simulink model "FP_Solutions_Part_3_disturbance"  (R2024b)
settings: Solver=VariableStepAuto  StartTime=0.0  StopTime=tspan  FixedStep=10  RelTol=1e-8
model workspace (MATLAB code in the model file):
  | mu = 398601; % km
  | Re = 6378.137; %km
values from neighbouring files (symbols this model uses):
  E_b_LVLH_0 = [phi_0; theta_0; psi_0]    [FP_Solution_Part_3.m]
  J = (Bus_I - Bus_m*skew(r_Bus)*skew(r_Bus)) +     (Sensor_I - Sensor_m*skew(r_Sensor)*skew(r_Sensor)) +      (Sp_minus_I - Sp_minus_m*skew(r_Sp_minus)*skew(r_Sp_minus)) +     (Sp_plus_I - Sp_plus_m*skew(r_Sp_plus)*skew(r_Sp_plus))    [FP_Solution_Part_3.m]
  JD_0 = 2460390    [FP_Solution_Part_3.m]
  q_b_LVLH_0 = [0; 0; 0; 1]    [FP_Solution_Part_3.m]
  residual_dipole_moment = [0;0;-0.5]    [FP_Solution_Part_3.m]
  Sun_vec = [1;0;0]    [FP_Solution_Part_3.m]
  surfaceProperties = [Areas rhos normals]    [FP_Solution_Part_3.m]
  T_c = [0; 0; 0]    [FP_Solution_Part_3.m]
undefined symbols (not defined in the file or in its folder): r_ECI_0, v_ECI_0
settings Model: Creator=emehiel  LastModifiedBy=nicho
settings SolverCC: AlgebraicLoopSolver=TrustRegion
settings DebuggingCC: UnconnectedInputMsg=warning  UnconnectedOutputMsg=warning  UnconnectedLineMsg=warning
settings ModelReferenceCC: EnableRefExpFcnMdlSchedulingChecks=on
settings RTWCC: GPUComputeCapability=3.5

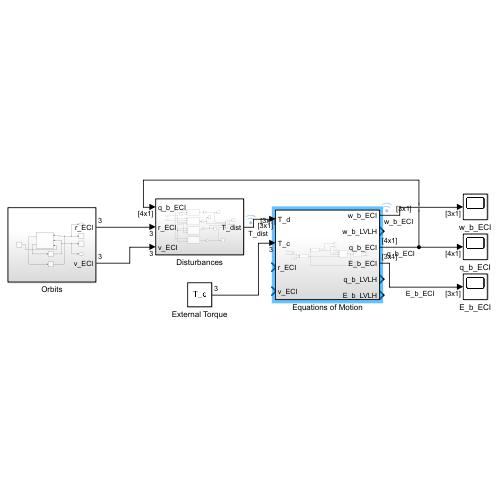
[thumbnail: Simulink's stored preview of the top-level diagram]
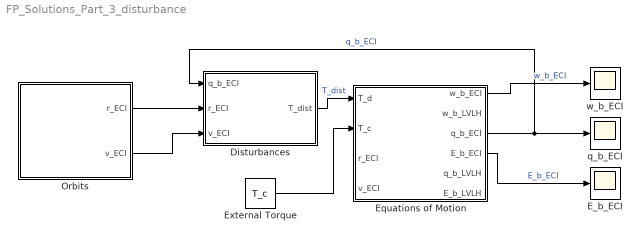
== system FP_Solutions_Part_3_disturbance ==
  Disturbances : Subsystem
  E_b_ECI : Scope
  Equations of Motion : Subsystem
  External Torque : Constant  Value=T_c
  Orbits : Subsystem
  q_b_ECI : Scope
  w_b_ECI : Scope
  wires:
  Orbits/1(r_ECI) -> Disturbances/2(r_ECI)
  Orbits/2(v_ECI) -> Disturbances/3(v_ECI)
  Equations of Motion/3(q_b_ECI) -> Disturbances/1(q_b_ECI), q_b_ECI/1  "q_b_ECI"
  Equations of Motion/1(w_b_ECI) -> w_b_ECI/1  "w_b_ECI"
  Disturbances/1(T_dist) -> Equations of Motion/1(T_d)  "T_dist"
  Equations of Motion/4(E_b_ECI) -> E_b_ECI/1  "E_b_ECI"
  External Torque/1 -> Equations of Motion/2(T_c)

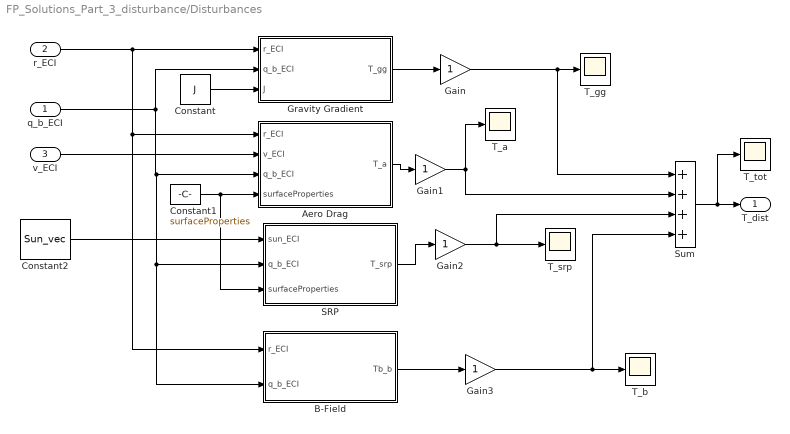
== system FP_Solutions_Part_3_disturbance/Disturbances ==
  q_b_ECI : Inport  PortDimensions=[4 1]
  r_ECI : Inport  Port=2
  v_ECI : Inport  Port=3
  Aero Drag : MATLAB Function  TreatAsAtomicUnit=on
  B-Field : Subsystem
  Constant : Constant  Value=J
  Constant1 : Constant  Value=surfaceProperties
  Constant2 : Constant  Value=Sun_vec
  Gain{,1..3} (4 alike) : Gain
  Gravity Gradient : MATLAB Function  TreatAsAtomicUnit=on
  SRP : MATLAB Function  TreatAsAtomicUnit=on
  Sum : Sum  Inputs=++++
  T_a : Scope
  T_b : Scope
  T_gg : Scope
  T_srp : Scope
  T_tot : Scope
  T_dist : Outport
  wires:
  Sum/1 -> T_tot/1, T_dist/1
  Aero Drag/1(T_a) -> Gain1/1
  Gravity Gradient/1(T_gg) -> Gain/1
  SRP/1(T_srp) -> Gain2/1
  Constant1/1 -> SRP/3(surfaceProperties), Aero Drag/4(surfaceProperties)
  v_ECI/1 -> Aero Drag/2(v_ECI)
  q_b_ECI/1 -> B-Field/2(q_b_ECI), SRP/2(q_b_ECI), Aero Drag/3(q_b_ECI), Gravity Gradient/2(q_b_ECI)
  Constant/1 -> Gravity Gradient/3(J)
  Constant2/1 -> SRP/1(sun_ECI)
  r_ECI/1 -> B-Field/1(r_ECI), Aero Drag/1(r_ECI), Gravity Gradient/1(r_ECI)
  B-Field/1(Tb_b) -> Gain3/1
  Gain/1 -> Sum/1, T_gg/1
  Gain1/1 -> Sum/2, T_a/1
  Gain3/1 -> T_b/1, Sum/4
  Gain2/1 -> Sum/3, T_srp/1

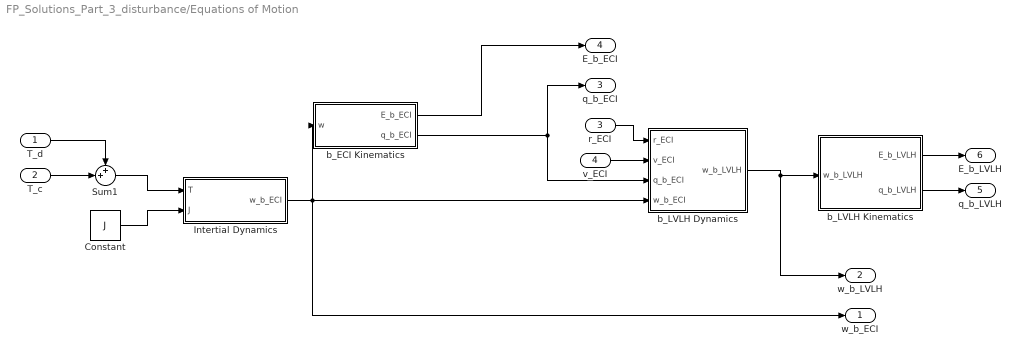
== system FP_Solutions_Part_3_disturbance/Equations of Motion ==
  T_d : Inport
  T_c : Inport  Port=2
  r_ECI : Inport  Port=3
  v_ECI : Inport  Port=4
  Constant : Constant  Value=J
  "Intertial Dynamics " : Subsystem
  Sum1 : Sum  Inputs=++|
  b_ECI Kinematics : Subsystem
  b_LVLH Dynamics : Subsystem
  b_LVLH Kinematics : Subsystem
  w_b_ECI : Outport  VectorParamsAs1DForOutWhenUnconnected=off
  w_b_LVLH : Outport  Port=2  PortDimensions=[3 1]  VectorParamsAs1DForOutWhenUnconnected=off
  q_b_ECI : Outport  Port=3  PortDimensions=[4 1]  VectorParamsAs1DForOutWhenUnconnected=off
  E_b_ECI : Outport  Port=4  PortDimensions=[3 1]  VectorParamsAs1DForOutWhenUnconnected=off
  q_b_LVLH : Outport  Port=5  PortDimensions=[4 1]  VectorParamsAs1DForOutWhenUnconnected=off
  E_b_LVLH : Outport  Port=6  PortDimensions=[3 1]  VectorParamsAs1DForOutWhenUnconnected=off
  wires:
  T_d/1 -> Sum1/1
  T_c/1 -> Sum1/2
  Sum1/1 -> "Intertial Dynamics "/1(T)
  Constant/1 -> "Intertial Dynamics "/2(J)
  b_ECI Kinematics/2(q_b_ECI) -> q_b_ECI/1, b_LVLH Dynamics/3(q_b_ECI)
  b_LVLH Kinematics/2(q_b_LVLH) -> q_b_LVLH/1
  r_ECI/1 -> b_LVLH Dynamics/1("r_ECI ")
  b_LVLH Dynamics/1(w_b_LVLH) -> w_b_LVLH/1, b_LVLH Kinematics/1(w_b_LVLH)
  "Intertial Dynamics "/1(w_b_ECI) -> w_b_ECI/1, b_LVLH Dynamics/4(w_b_ECI), b_ECI Kinematics/1(w)
  b_ECI Kinematics/1(E_b_ECI) -> E_b_ECI/1
  v_ECI/1 -> b_LVLH Dynamics/2(v_ECI)
  b_LVLH Kinematics/1(E_b_LVLH) -> E_b_LVLH/1

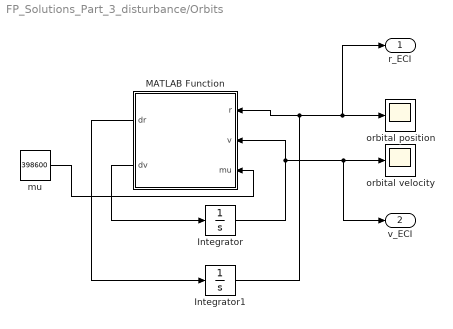
== system FP_Solutions_Part_3_disturbance/Orbits ==
  Integrator : Integrator  InitialCondition=v_ECI_0
  Integrator1 : Integrator  InitialCondition=r_ECI_0
  MATLAB Function : MATLAB Function  TreatAsAtomicUnit=on
  mu : Constant  Value=398600
  orbital position : Scope
  orbital velocity : Scope
  r_ECI : Outport  VectorParamsAs1DForOutWhenUnconnected=off
  v_ECI : Outport  Port=2  VectorParamsAs1DForOutWhenUnconnected=off
  wires:
  Integrator/1 -> v_ECI/1, orbital velocity/1, MATLAB Function/2(v)
  Integrator1/1 -> r_ECI/1, orbital position/1, MATLAB Function/1(r)
  MATLAB Function/1(dr) -> Integrator1/1
  MATLAB Function/2(dv) -> Integrator/1
  mu/1 -> MATLAB Function/3(mu)

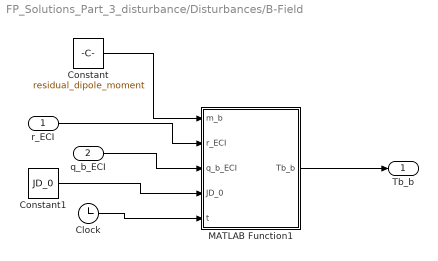
== system FP_Solutions_Part_3_disturbance/Disturbances/B-Field ==
  r_ECI : Inport
  q_b_ECI : Inport  Port=2
  Clock : Clock
  Constant : Constant  Value=residual_dipole_moment  VectorParams1D=off
  Constant1 : Constant  Value=JD_0
  MATLAB Function1 : MATLAB Function  TreatAsAtomicUnit=on
  Tb_b : Outport
  wires:
  MATLAB Function1/1(Tb_b) -> Tb_b/1
  q_b_ECI/1 -> MATLAB Function1/3(q_b_ECI)
  r_ECI/1 -> MATLAB Function1/2(r_ECI)
  Clock/1 -> MATLAB Function1/5(t)
  Constant1/1 -> MATLAB Function1/4(JD_0)
  Constant/1 -> MATLAB Function1/1(m_b)

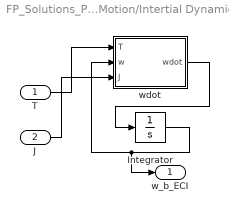
== system FP_Solutions_Part_3_disturbance/Equations of Motion/Intertial Dynamics  ==
  T : Inport
  J : Inport  Port=2
  Integrator : Integrator  InitialCondition=[0.001; -0.001; 0.002]
  wdot : MATLAB Function  TreatAsAtomicUnit=on
  w_b_ECI : Outport
  wires:
  Integrator/1 -> wdot/2(w), w_b_ECI/1
  wdot/1(wdot) -> Integrator/1
  T/1 -> wdot/1(T)
  J/1 -> wdot/3(J)

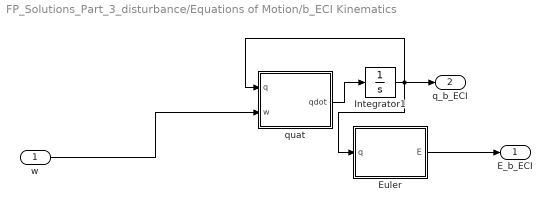
== system FP_Solutions_Part_3_disturbance/Equations of Motion/b_ECI Kinematics ==
  w : Inport
  Euler : MATLAB Function  TreatAsAtomicUnit=on
  Integrator1 : Integrator  InitialCondition=[0;0;0;1]
  quat : MATLAB Function  TreatAsAtomicUnit=on
  E_b_ECI : Outport  VectorParamsAs1DForOutWhenUnconnected=off
  q_b_ECI : Outport  Port=2  VectorParamsAs1DForOutWhenUnconnected=off
  wires:
  w/1 -> quat/2(w)
  Integrator1/1 -> quat/1(q), Euler/1(q), q_b_ECI/1
  quat/1(qdot) -> Integrator1/1
  Euler/1(E) -> E_b_ECI/1

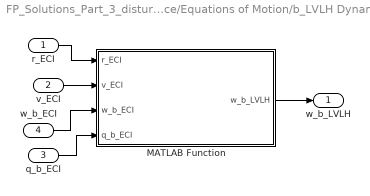
== system FP_Solutions_Part_3_disturbance/Equations of Motion/b_LVLH Dynamics ==
  "r_ECI " : Inport
  v_ECI : Inport  Port=2
  q_b_ECI : Inport  Port=3
  w_b_ECI : Inport  Port=4
  MATLAB Function : MATLAB Function  TreatAsAtomicUnit=on
  w_b_LVLH : Outport  VectorParamsAs1DForOutWhenUnconnected=off
  wires:
  MATLAB Function/1(w_b_LVLH) -> w_b_LVLH/1
  "r_ECI "/1 -> MATLAB Function/1(r_ECI)
  v_ECI/1 -> MATLAB Function/2(v_ECI)
  q_b_ECI/1 -> MATLAB Function/4(q_b_ECI)
  w_b_ECI/1 -> MATLAB Function/3(w_b_ECI)

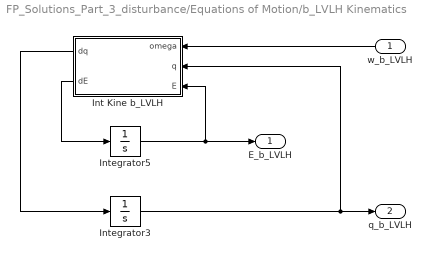
== system FP_Solutions_Part_3_disturbance/Equations of Motion/b_LVLH Kinematics ==
  w_b_LVLH : Inport
  Int Kine b_LVLH : MATLAB Function  TreatAsAtomicUnit=on
  Integrator3 : Integrator  InitialCondition=q_b_LVLH_0
  Integrator5 : Integrator  InitialCondition=E_b_LVLH_0
  E_b_LVLH : Outport  PortDimensions=[3 1]  VectorParamsAs1DForOutWhenUnconnected=off
  q_b_LVLH : Outport  Port=2  VectorParamsAs1DForOutWhenUnconnected=off
  wires:
  Int Kine b_LVLH/1(dq) -> Integrator3/1
  Integrator3/1 -> Int Kine b_LVLH/2(q), q_b_LVLH/1
  Int Kine b_LVLH/2(dE) -> Integrator5/1
  Integrator5/1 -> E_b_LVLH/1, Int Kine b_LVLH/3(E)
  w_b_LVLH/1 -> Int Kine b_LVLH/1(omega)

== matlab function FP_Solutions_Part_3_disturbance/Equations of Motion/b_ECI Kinematics/quat ==
  data: q input; qdot output; w input
function qdot = fcn(q, w)
%#codegen

q = reshape(q,4,1);
w = reshape(w,3,1);

wx = w(1);
wy = w(2);
wz = w(3);

Omega = [  0   -wx  -wy  -wz;
          wx    0    wz  -wy;
          wy   -wz   0    wx;
          wz    wy  -wx   0 ];

qdot = 0.5 * Omega * q;

end

== matlab function FP_Solutions_Part_3_disturbance/Equations of Motion/b_LVLH Dynamics/MATLAB Function ==
  data: r_ECI input; v_ECI input; w_b_ECI input; q_b_ECI input; w_b_LVLH output
function w_b_LVLH = fcn(r_ECI, v_ECI, w_b_ECI, q_b_ECI)
%#codegen

% Compute the angular velocity of LVLH wrt ECI in Body components

rhat = r_ECI / norm(r_ECI);
hvec = cross(r_ECI, v_ECI);
hhat = hvec / norm(hvec);
that = cross(-rhat, hhat);
that = that / norm(that);

C_LVLH_ECI = [hhat.';
                that.';
               (-rhat).'];

q_b_LVLH = circle_cross(transpose(C_LVLH_ECI),q_b_ECI);

w_b_LVLH = w_b_ECI*transpose(C_LVLH_ECI);

== matlab function FP_Solutions_Part_3_disturbance/Disturbances/Gravity Gradient ==
  data: r_ECI input; T_gg output; q_b_ECI input; J input
function T_gg = gg_torque(r_ECI, q_b_ECI, J)
% GG_TORQUE Gravity-gradient torque in body frame
%
% Inputs:
%   r_ECI    3x1 position vector in ECI [km]
%   q_b_ECI  4x1 quaternion [q1;q2;q3;q4], scalar last
%   J        3x3 spacecraft inertia matrix [kg*m^2]
%
% Output:
%   T_gg     3x1 gravity-gradient torque in body frame [N*m]

    mu = 398600;  % km^3/s^2

    r_ECI = r_ECI(:);
    q_b_ECI = q_b_ECI(:);

    r = norm(r_ECI);
    if r == 0
        T_gg = zeros(3,1);
        return
    end

    % Position direction in body frame
    C_b_ECI = quat2C(q_b_ECI);
    r_b = C_b_ECI * r_ECI;
    rhat_b = r_b / norm(r_b);

    % Gravity-gradient torque
    T_gg = (3*mu/r^5) * cross(rhat_b, J*rhat_b);
end

== matlab function FP_Solutions_Part_3_disturbance/Disturbances/Aero Drag ==
  data: r_ECI input; v_ECI input; T_a output; q_b_ECI input; surfaceProperties input
function T_a = aero_drag_torque(r_ECI, v_ECI, q_b_ECI, surfaceProperties)
% AERO_DRAG_TORQUE Atmospheric drag torque in body frame
%
% Inputs:
%   r_ECI            3x1 position in ECI [km]
%   v_ECI            3x1 velocity in ECI [km/s]
%   q_b_ECI          4x1 quaternion [q1;q2;q3;q4], scalar last
%   surfaceProperties Nx7 matrix:
%                     col 1   = area
%                     col 2:4 = center of pressure in body frame
%                     col 5:7 = surface normal in body frame
%
% Output:
%   T_a              3x1 aerodynamic drag torque in body frame [N*m]

    % Constants
    Cd = 2.2;                 % drag coefficient
    rho0 = 1.225;             % sea-level density [kg/m^3]
    H = 8500;                 % scale height [m]
    R_E = 6378e3;             % Earth radius [m]

    % Force column vectors
    r_ECI = r_ECI(:);
    v_ECI = v_ECI(:);
    q_b_ECI = q_b_ECI(:);

    % Initialize output
    T_a = zeros(3,1);

    % Convert ECI state to SI units
    r_m = 1000 * r_ECI;       % [m]
    v_m = 1000 * v_ECI;       % [m/s]

    % Convert velocity from ECI to body
    C_b_ECI = quat2C(q_b_ECI);
    v_b = C_b_ECI * v_m;

    % Relative wind direction is opposite velocity
    vmag = norm(v_b);
    if vmag == 0
        return
    end

    vhat_b = v_b / vmag;
    flow_dir = -vhat_b;

    % Simple exponential atmosphere model
    alt = norm(r_m) - R_E;
    rho = rho0 * exp(-alt / H);

    % Loop through all spacecraft surfaces
    nSurf = size(surfaceProperties,1);

    for i = 1:nSurf
        A   = surfaceProperties(i,1);
        rho_cp = surfaceProperties(i,2:4).';   % center of pressure in body
        n   = surfaceProperties(i,5:7).';      % outward normal in body

        if norm(n) == 0
            continue
        end
        n = n / norm(n);

        % Wetted projected area
        A_wet = A * dot(n, flow_dir);

        if A_wet > 0
            % Drag force on this surface
            F_a = 0.5 * rho * Cd * vmag^2 * A_wet * flow_dir;

            % Add torque contribution
            T_a = T_a + cross(rho_cp, F_a);
        end
    end
end

== matlab function FP_Solutions_Part_3_disturbance/Disturbances/SRP ==
  data: sun_ECI input; T_srp output; q_b_ECI input; surfaceProperties input
function T_srp = SPR_torque(sun_ECI, q_b_ECI, surfaceProperties)
%#codegen

p_sun = 4.5e-6; % N/m^2

sun_ECI = sun_ECI(:);
q_b_ECI = q_b_ECI(:);

T_srp = zeros(3,1);

C_b_ECI = quat2C(q_b_ECI);
sun_b = C_b_ECI * sun_ECI;

sun_norm = norm(sun_b);
if sun_norm == 0
    return
end
sun_b = sun_b / sun_norm;

nSurf = size(surfaceProperties,1);

for k = 1:nSurf
    A = surfaceProperties(k,1);
    rho_cp = surfaceProperties(k,2:4).';
    n = surfaceProperties(k,5:7).';

    n_norm = norm(n);
    if n_norm == 0
        continue
    end
    n = n / n_norm;

    ctheta = dot(n, sun_b);

    if ctheta > 0
        F_srp = -p_sun * A * ctheta * sun_b;
        T_srp = T_srp + cross(rho_cp, F_srp);
    end
end

end

== matlab function FP_Solutions_Part_3_disturbance/Orbits/MATLAB Function ==
  data: r input; dr output; v input; dv output; mu input
function [dr, dv] = f(r, v, mu)
%#codegen

% Force column vectors
r = r(:);
v = v(:);

% Preallocate outputs
dr = zeros(3,1);
dv = zeros(3,1);

rnorm = norm(r);

dr = v;
dv = -(mu / rnorm^3) * r;
end

== matlab function FP_Solutions_Part_3_disturbance/Disturbances/B-Field/MATLAB Function1 ==
  data: m_b input; r_ECI input; q_b_ECI input; Tb_b output; JD_0 input; t input
function Tb_b = WMM(m_b, r_ECI, q_b_ECI, JD_0, t)
%#codegen

Tb_b = zeros(3,1);

m_b = m_b(:);
r_ECI = r_ECI(:);
q_b_ECI = q_b_ECI(:);

end

== matlab function FP_Solutions_Part_3_disturbance/Equations of Motion/b_ECI Kinematics/Euler ==
  data: q input; E output
function E = fcn(q)
%#codegen

q = reshape(q,4,1);
C = quat2C(q);
E = C2EulerAngles(C);
E = reshape(E,3,1);

end

== matlab function FP_Solutions_Part_3_disturbance/Equations of Motion/Intertial Dynamics /wdot ==
  data: T input size=[3 1]; w input size=[3 1]; wdot output size=[3 1]; J input size=[3 3]
function wdot = fcn(T, w, J)
%#codegen

wdot = J\ (T - cross(w, J*w));

end

== matlab function FP_Solutions_Part_3_disturbance/Equations of Motion/b_LVLH Kinematics/Int Kine b_LVLH ==
  data: omega input; q input; dq output; E input; dE output
function [dq,dE] = kinematics(omega, q, E)
%#codegen

% unpack quaternion

% compute the derivative of the quaternion components here

% compute the derivative of the Euler Angle components here
